simulink model "simulator_model"  (R2016a)
settings: Solver=FixedStepAuto  StartTime=0.0  StopTime=30  FixedStep=0.1  RelTol=1e-3
model workspace: external: MAT-File /home/combine/bin/ExjobbROV/simulink/Estimation/parameters.mat (data not in the file)
libraries: simulink x10, dspsrcs4 x6
settings Model: SimulationMode=accelerator  Creator=erik  LastModifiedBy=combine
settings DataIOCC: LimitDataPoints=on  InspectSignalLogs=on
settings OptimizationCC: EfficientMapNaN2IntZero=off
settings DebuggingCC: AllowSymbolicDim=off
settings HardwareCC: TargetBitPerLong=64  TargetBitPerPointer=64  TargetLongLongMode=on  TargetIntDivRoundTo=Zero  TargetEndianess=LittleEndian  TargetWordSize=64  TargetHWDeviceType=MATLAB Host  ProdEqTarget=off
settings ModelReferenceCC: PropagateSignalLabelsOutOfModel=off
settings CodeAppCC: MaxIdLength=128
settings GRTTargetCC: GeneratePreprocessorConditionals=Use local settings  CombineOutputUpdateFcns=off  GRTInterface=on

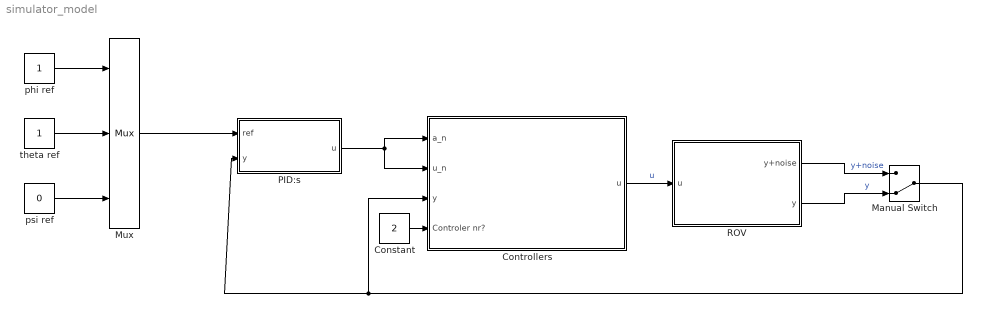
== system simulator_model ==
  Constant : Constant  Value=2
  Controllers : Subsystem
  Manual Switch : ManualSwitch  CurrentSetting=0
  Mux : Mux  Inputs=3
  PID:s : Subsystem
  ROV : Subsystem
  phi ref : Constant
  "psi ref " : Constant  Value=0
  "theta ref " : Constant
  wires:
  Controllers/1(u) -> ROV/1(u)  "u"
  Constant/1 -> Controllers/4(Controler nr?)
  ROV/2(y) -> Manual Switch/2  "y"
  ROV/1(y+noise) -> Manual Switch/1  "y+noise"
  Manual Switch/1 -> PID:s/2(y), Controllers/3(y)
  PID:s/1(u) -> Controllers/2(u_n), Controllers/1(a_n)
  phi ref/1 -> Mux/1
  "theta ref "/1 -> Mux/2
  "psi ref "/1 -> Mux/3
  Mux/1 -> PID:s/1(ref)

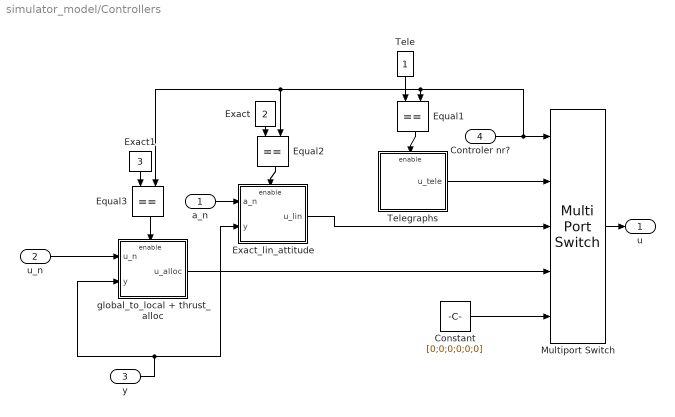
== system simulator_model/Controllers ==
  a_n : Inport
  u_n : Inport  Port=2
  y : Inport  Port=3
  Controler nr? : Inport  Port=4
  Constant : Constant  Value=[0;0;0;0;0;0]
  Equal1 : RelationalOperator  Operator===  OutDataTypeStr=boolean
  Equal2 : RelationalOperator  Operator===  OutDataTypeStr=boolean
  Equal3 : RelationalOperator  Operator===  OutDataTypeStr=boolean
  Exact : Constant  Value=2
  Exact1 : Constant  Value=3
  Exact_lin_attitude : Subsystem
  Multiport Switch : MultiPortSwitch  Inputs=4
  Tele : Constant
  Telegraphs : Subsystem
  global_to_local + thrust_alloc : Subsystem
  u : Outport
  wires:
  Exact1/1 -> Equal3/1
  Multiport Switch/1 -> u/1
  Constant/1 -> Multiport Switch/5
  Telegraphs/1(u_tele) -> Multiport Switch/2
  Exact_lin_attitude/1(u_lin) -> Multiport Switch/3
  global_to_local + thrust_alloc/1(u_alloc) -> Multiport Switch/4
  Controler nr?/1 -> Multiport Switch/1, Equal1/2, Equal2/2, Equal3/2
  Equal1/1 -> Telegraphs/Enable
  Tele/1 -> Equal1/1
  Exact/1 -> Equal2/1
  Equal2/1 -> Exact_lin_attitude/Enable
  Equal3/1 -> global_to_local + thrust_alloc/Enable
  y/1 -> Exact_lin_attitude/2(y), global_to_local + thrust_alloc/2(y)
  u_n/1 -> global_to_local + thrust_alloc/1(u_n)
  a_n/1 -> Exact_lin_attitude/1(a_n)

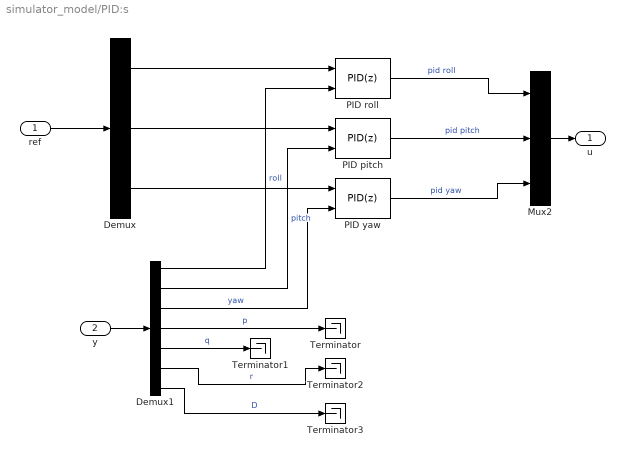
== system simulator_model/PID:s ==
  ref : Inport
  y : Inport  Port=2
  Demux : Demux  Outputs=3
  Demux1 : Demux  Outputs=7
  Mux2 : Mux  Inputs=3
  PID pitch : simulink/Continuous/PID Controller (2DOF)  Controller=PID  TimeDomain=Discrete-time  SampleTime=-1  IntegratorMethod=Forward Euler  FilterMethod=Forward Euler  Form=Parallel  UseFilter=on  ControllerParametersSource=internal  P=1  I=1  D=0  N=1  b=1  c=1  InitialConditionSource=internal  InitialConditionForIntegrator=0  InitialConditionForFilter=0  ExternalReset=none  LimitOutput=off  UpperSaturationLimit=inf  LowerSaturationLimit=-inf  LinearizeAsGain=on  AntiWindupMode=none  Kb=1  TrackingMode=off  Kt=1  PParamMin=[]  PParamMax=[]  IParamMin=[]  IParamMax=[]  DParamMin=[]  DParamMax=[]  NParamMin=[]  NParamMax=[]  bParamMin=[]  bParamMax=[]  cParamMin=[]  cParamMax=[]  KbParamMin=[]  KbParamMax=[]  KtParamMin=[]  KtParamMax=[]  POutMin=[]  POutMax=[]  IOutMin=[]  IOutMax=[]  DOutMin=[]  DOutMax=[]  NOutMin=[]  NOutMax=[]  bOutMin=[]  bOutMax=[]  cOutMin=[]  cOutMax=[]  KbOutMin=[]  KbOutMax=[]  KtOutMin=[]  KtOutMax=[]  IntegratorOutMin=[]  IntegratorOutMax=[]  FilterOutMin=[]  FilterOutMax=[]  SumOutMin=[]  SumOutMax=[]  Sum1OutMin=[]  Sum1OutMax=[]  Sum2OutMin=[]  Sum2OutMax=[]  Sum3OutMin=[]  Sum3OutMax=[]  SumI1OutMin=[]  SumI1OutMax=[]  SumI2OutMin=[]  SumI2OutMax=[]  SumI3OutMin=[]  SumI3OutMax=[]  SumDOutMin=[]  SumDOutMax=[]  SaturationOutMin=[]  SaturationOutMax=[]  IntegratorContinuousStateAttributes=''  IntegratorStateMustResolveToSignalObject=off  IntegratorRTWStateStorageClass=Auto  FilterContinuousStateAttributes=''  FilterStateMustResolveToSignalObject=off  FilterRTWStateStorageClass=Auto  DifferentiatorICPrevScaledInput=0  DifferentiatorOutMin=[]  DifferentiatorOutMax=[]
  PID roll : simulink/Continuous/PID Controller (2DOF)  Controller=PID  TimeDomain=Discrete-time  SampleTime=-1  IntegratorMethod=Forward Euler  FilterMethod=Forward Euler  Form=Parallel  UseFilter=on  ControllerParametersSource=internal  P=1  I=1  D=0  N=1  b=1  c=1  InitialConditionSource=internal  InitialConditionForIntegrator=0  InitialConditionForFilter=0  ExternalReset=none  LimitOutput=off  UpperSaturationLimit=inf  LowerSaturationLimit=-inf  LinearizeAsGain=on  AntiWindupMode=none  Kb=1  TrackingMode=off  Kt=1  PParamMin=[]  PParamMax=[]  IParamMin=[]  IParamMax=[]  DParamMin=[]  DParamMax=[]  NParamMin=[]  NParamMax=[]  bParamMin=[]  bParamMax=[]  cParamMin=[]  cParamMax=[]  KbParamMin=[]  KbParamMax=[]  KtParamMin=[]  KtParamMax=[]  POutMin=[]  POutMax=[]  IOutMin=[]  IOutMax=[]  DOutMin=[]  DOutMax=[]  NOutMin=[]  NOutMax=[]  bOutMin=[]  bOutMax=[]  cOutMin=[]  cOutMax=[]  KbOutMin=[]  KbOutMax=[]  KtOutMin=[]  KtOutMax=[]  IntegratorOutMin=[]  IntegratorOutMax=[]  FilterOutMin=[]  FilterOutMax=[]  SumOutMin=[]  SumOutMax=[]  Sum1OutMin=[]  Sum1OutMax=[]  Sum2OutMin=[]  Sum2OutMax=[]  Sum3OutMin=[]  Sum3OutMax=[]  SumI1OutMin=[]  SumI1OutMax=[]  SumI2OutMin=[]  SumI2OutMax=[]  SumI3OutMin=[]  SumI3OutMax=[]  SumDOutMin=[]  SumDOutMax=[]  SaturationOutMin=[]  SaturationOutMax=[]  IntegratorContinuousStateAttributes=''  IntegratorStateMustResolveToSignalObject=off  IntegratorRTWStateStorageClass=Auto  FilterContinuousStateAttributes=''  FilterStateMustResolveToSignalObject=off  FilterRTWStateStorageClass=Auto  DifferentiatorICPrevScaledInput=0  DifferentiatorOutMin=[]  DifferentiatorOutMax=[]
  PID yaw : simulink/Continuous/PID Controller (2DOF)  Controller=PID  TimeDomain=Discrete-time  SampleTime=-1  IntegratorMethod=Forward Euler  FilterMethod=Forward Euler  Form=Parallel  UseFilter=on  ControllerParametersSource=internal  P=0  I=0  D=0  N=1  b=1  c=1  InitialConditionSource=internal  InitialConditionForIntegrator=0  InitialConditionForFilter=0  ExternalReset=none  LimitOutput=off  UpperSaturationLimit=inf  LowerSaturationLimit=-inf  LinearizeAsGain=on  AntiWindupMode=none  Kb=1  TrackingMode=off  Kt=1  PParamMin=[]  PParamMax=[]  IParamMin=[]  IParamMax=[]  DParamMin=[]  DParamMax=[]  NParamMin=[]  NParamMax=[]  bParamMin=[]  bParamMax=[]  cParamMin=[]  cParamMax=[]  KbParamMin=[]  KbParamMax=[]  KtParamMin=[]  KtParamMax=[]  POutMin=[]  POutMax=[]  IOutMin=[]  IOutMax=[]  DOutMin=[]  DOutMax=[]  NOutMin=[]  NOutMax=[]  bOutMin=[]  bOutMax=[]  cOutMin=[]  cOutMax=[]  KbOutMin=[]  KbOutMax=[]  KtOutMin=[]  KtOutMax=[]  IntegratorOutMin=[]  IntegratorOutMax=[]  FilterOutMin=[]  FilterOutMax=[]  SumOutMin=[]  SumOutMax=[]  Sum1OutMin=[]  Sum1OutMax=[]  Sum2OutMin=[]  Sum2OutMax=[]  Sum3OutMin=[]  Sum3OutMax=[]  SumI1OutMin=[]  SumI1OutMax=[]  SumI2OutMin=[]  SumI2OutMax=[]  SumI3OutMin=[]  SumI3OutMax=[]  SumDOutMin=[]  SumDOutMax=[]  SaturationOutMin=[]  SaturationOutMax=[]  IntegratorContinuousStateAttributes=''  IntegratorStateMustResolveToSignalObject=off  IntegratorRTWStateStorageClass=Auto  FilterContinuousStateAttributes=''  FilterStateMustResolveToSignalObject=off  FilterRTWStateStorageClass=Auto  DifferentiatorICPrevScaledInput=0  DifferentiatorOutMin=[]  DifferentiatorOutMax=[]
  Terminator{,1..3} (4 alike) : Terminator
  u : Outport
  wires:
  Mux2/1 -> u/1
  Demux1/1 -> PID roll/2  "roll"
  Demux1/2 -> PID pitch/2  "pitch"
  Demux1/3 -> PID yaw/2  "yaw"
  Demux/2 -> PID pitch/1
  PID pitch/1 -> Mux2/2  "pid pitch"
  Demux/1 -> PID roll/1
  PID roll/1 -> Mux2/1  "pid roll"
  PID yaw/1 -> Mux2/3  "pid yaw"
  Demux/3 -> PID yaw/1
  y/1 -> Demux1/1
  ref/1 -> Demux/1
  Demux1/4 -> Terminator/1  "p"
  Demux1/5 -> Terminator1/1  "q"
  Demux1/6 -> Terminator2/1  "r"
  Demux1/7 -> Terminator3/1  "D"

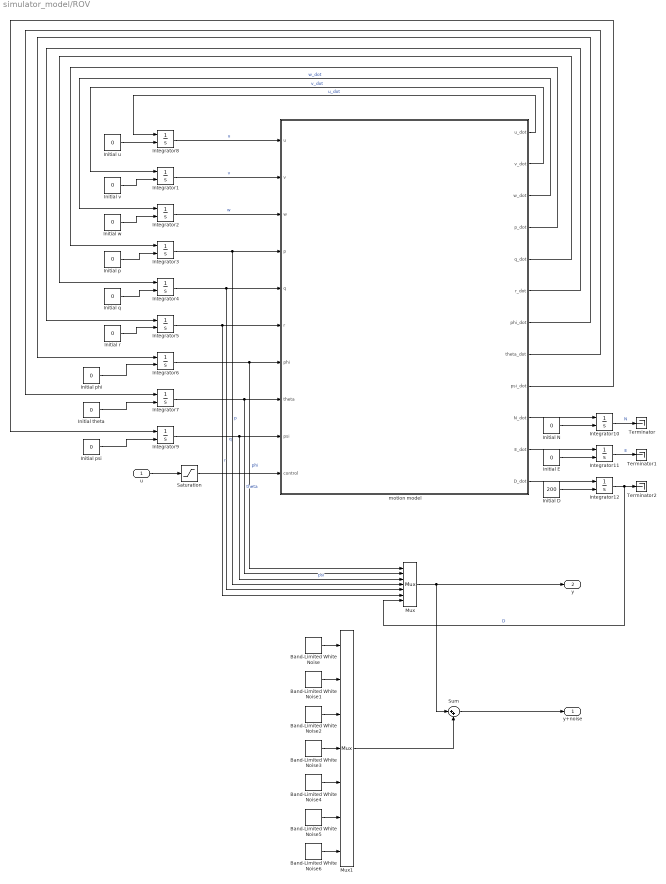
== system simulator_model/ROV ==
  u : Inport
  Band-Limited White Noise : simulink/Sources/Band-Limited White Noise  Cov=0.0005  Ts=0.1  seed=[23341]
  Band-Limited White Noise1 : simulink/Sources/Band-Limited White Noise  Cov=0.0005  Ts=0.1  seed=[29023]
  Band-Limited White Noise2 : simulink/Sources/Band-Limited White Noise  Cov=0.0005  Ts=0.1  seed=[91318]
  Band-Limited White Noise3 : simulink/Sources/Band-Limited White Noise  Cov=0.0005  Ts=0.1  seed=[2333451]
  Band-Limited White Noise4 : simulink/Sources/Band-Limited White Noise  Cov=0.0005  Ts=0.1  seed=[21241]
  Band-Limited White Noise5 : simulink/Sources/Band-Limited White Noise  Cov=0.0005  Ts=0.1  seed=[12345]
  Band-Limited White Noise6 : simulink/Sources/Band-Limited White Noise  Cov=0.0005  Ts=0.1  seed=[9875]
  Initial D : Constant  Value=200
  Initial E : Constant  Value=0
  Initial N : Constant  Value=0
  Initial p : Constant  Value=0
  Initial phi : Constant  Value=0
  Initial psi : Constant  Value=0
  Initial q : Constant  Value=0
  Initial r : Constant  Value=0
  Initial theta : Constant  Value=0
  Initial u : Constant  Value=0
  Initial v : Constant  Value=0
  Initial w : Constant  Value=0
  Integrator{1..12} (12 alike) : Integrator  InitialConditionSource=external
  Mux : Mux  Inputs=7
  Mux1 : Mux  Inputs=7
  Saturation : Saturate  UpperLimit=1  LowerLimit=-1
  Sum : Sum  Inputs=|++
  Terminator : Terminator
  Terminator1 : Terminator
  Terminator2 : Terminator
  motion model : MATLAB Function  TreatAsAtomicUnit=on
  y+noise : Outport  PortDimensions=7
  y : Outport  Port=2  PortDimensions=7
  wires:
  u/1 -> Saturation/1
  Integrator8/1 -> motion model/1(u)  "u"
  Integrator1/1 -> motion model/2(v)  "v"
  Integrator2/1 -> motion model/3(w)  "w"
  Integrator3/1 -> Mux/4, motion model/4(p)  "p"
  Integrator4/1 -> Mux/5, motion model/5(q)  "q"
  Integrator5/1 -> Mux/6, motion model/6(r)  "r"
  Integrator7/1 -> Mux/2, motion model/8(theta)  "theta"
  Integrator9/1 -> Mux/3, motion model/9(psi)  "psi"
  motion model/1(u_dot) -> Integrator8/1  "u_dot"
  motion model/2(v_dot) -> Integrator1/1  "v_dot"
  motion model/3(w_dot) -> Integrator2/1  "w_dot"
  motion model/4(p_dot) -> Integrator3/1
  motion model/5(q_dot) -> Integrator4/1
  motion model/6(r_dot) -> Integrator5/1
  motion model/7(phi_dot) -> Integrator6/1
  motion model/8(theta_dot) -> Integrator7/1
  motion model/9(psi_dot) -> Integrator9/1
  Initial u/1 -> Integrator8/2
  Initial v/1 -> Integrator1/2
  Initial w/1 -> Integrator2/2
  Initial p/1 -> Integrator3/2
  Initial q/1 -> Integrator4/2
  Initial r/1 -> Integrator5/2
  Initial phi/1 -> Integrator6/2
  Integrator6/1 -> Mux/1, motion model/7(phi)  "phi"
  Initial theta/1 -> Integrator7/2
  Initial psi/1 -> Integrator9/2
  motion model/10(N_dot) -> Integrator10/1
  motion model/11(E_dot) -> Integrator11/1
  motion model/12(D_dot) -> Integrator12/1
  Initial E/1 -> Integrator11/2
  Initial N/1 -> Integrator10/2
  Initial D/1 -> Integrator12/2
  Integrator10/1 -> Terminator/1  "N"
  Integrator11/1 -> Terminator1/1  "E"
  Integrator12/1 -> Mux/7, Terminator2/1  "D"
  Mux/1 -> Sum/1, y/1
  Sum/1 -> y+noise/1
  Saturation/1 -> motion model/10(control)
  Band-Limited White Noise/1 -> Mux1/1
  Band-Limited White Noise1/1 -> Mux1/2
  Band-Limited White Noise2/1 -> Mux1/3
  Band-Limited White Noise3/1 -> Mux1/4
  Band-Limited White Noise4/1 -> Mux1/5
  Band-Limited White Noise5/1 -> Mux1/6
  Band-Limited White Noise6/1 -> Mux1/7
  Mux1/1 -> Sum/2

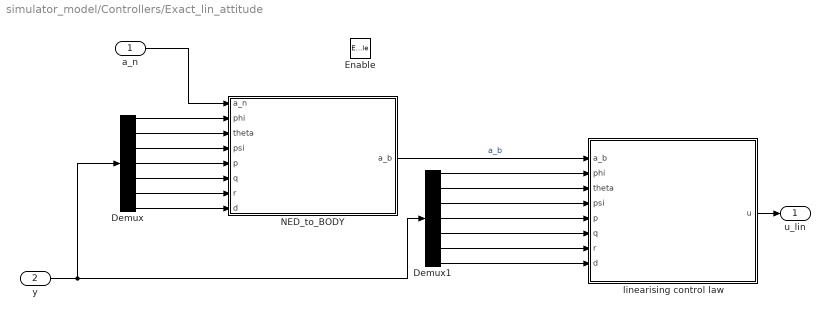
== system simulator_model/Controllers/Exact_lin_attitude ==
  a_n : Inport  PortDimensions=3
  y : Inport  Port=2  PortDimensions=7
  Enable : EnablePort
  Demux : Demux  Outputs=7
  Demux1 : Demux  Outputs=7
  NED_to_BODY : MATLAB Function  TreatAsAtomicUnit=on
  linearising control law : MATLAB Function  TreatAsAtomicUnit=on
  u_lin : Outport  PortDimensions=6
  wires:
  linearising control law/1(u) -> u_lin/1
  a_n/1 -> NED_to_BODY/1(a_n)
  NED_to_BODY/1(a_b) -> linearising control law/1(a_b)  "a_b"
  y/1 -> Demux1/1, Demux/1
  Demux/6 -> NED_to_BODY/7(r)
  Demux/4 -> NED_to_BODY/5(p)
  Demux/7 -> NED_to_BODY/8(d)
  Demux/1 -> NED_to_BODY/2(phi)
  Demux/3 -> NED_to_BODY/4(psi)
  Demux/5 -> NED_to_BODY/6(q)
  Demux/2 -> NED_to_BODY/3(theta)
  Demux1/1 -> linearising control law/2(phi)
  Demux1/2 -> linearising control law/3(theta)
  Demux1/3 -> linearising control law/4(psi)
  Demux1/4 -> linearising control law/5(p)
  Demux1/5 -> linearising control law/6(q)
  Demux1/6 -> linearising control law/7(r)
  Demux1/7 -> linearising control law/8(d)

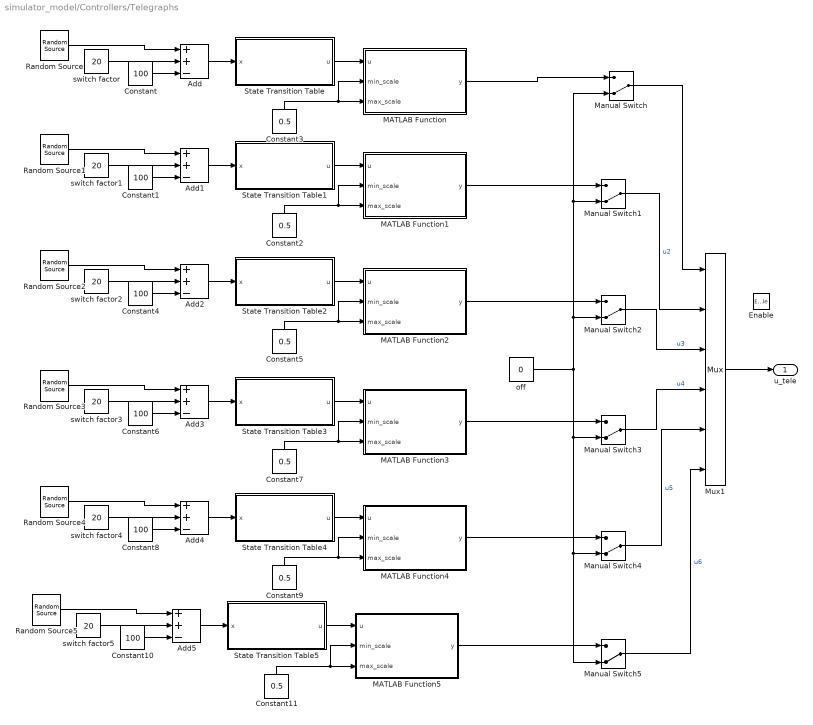
== system simulator_model/Controllers/Telegraphs ==
  Enable : EnablePort
  Add{,1..5} (6 alike) : Sum  Inputs=++-
  Constant{,1,4,6,8,10} (6 alike) : Constant  Value=100
  Constant{2..3,5,7,9,11} (6 alike) : Constant  Value=0.5
  MATLAB Function : MATLAB Function  TreatAsAtomicUnit=on
  MATLAB Function1 : MATLAB Function  TreatAsAtomicUnit=on
  MATLAB Function2 : MATLAB Function  TreatAsAtomicUnit=on
  MATLAB Function3 : MATLAB Function  TreatAsAtomicUnit=on
  MATLAB Function4 : MATLAB Function  TreatAsAtomicUnit=on
  MATLAB Function5 : MATLAB Function  TreatAsAtomicUnit=on
  Manual Switch{,1..5} (6 alike) : ManualSwitch  CurrentSetting=0
  Mux1 : Mux  Inputs=6
  Random Source{,1..5} (6 alike) : dspsrcs4/Random Source  SrcType=Uniform  NormMethod=Ziggurat  CltLength=12  MinVal=1  MaxVal=100  MeanVal=0  VarVal=1  RepMode=Not repeatable  rawSeed=1  IsInherit=on  SampMode=Discrete  SampTime=0.1  SampFrame=1  DataType=Double  OutComplex=Real  OutputFrames=off
  State Transition Table : State Transition Table  TreatAsAtomicUnit=on
  State Transition Table1 : State Transition Table  TreatAsAtomicUnit=on
  State Transition Table2 : State Transition Table  TreatAsAtomicUnit=on
  State Transition Table3 : State Transition Table  TreatAsAtomicUnit=on
  State Transition Table4 : State Transition Table  TreatAsAtomicUnit=on
  State Transition Table5 : State Transition Table  TreatAsAtomicUnit=on
  off : Constant  Value=0
  switch factor{,1..5} (6 alike) : Constant  Value=20
  u_tele : Outport
  wires:
  Random Source/1 -> Add/1
  Constant/1 -> Add/3
  Add/1 -> State Transition Table/1(x)
  switch factor/1 -> Add/2
  State Transition Table/1(u) -> MATLAB Function/1(u)
  Constant3/1 -> MATLAB Function/3(max_scale), MATLAB Function/2(min_scale)
  Random Source1/1 -> Add1/1
  Constant1/1 -> Add1/3
  Add1/1 -> State Transition Table1/1(x)
  switch factor1/1 -> Add1/2
  State Transition Table1/1(u) -> MATLAB Function1/1(u)
  Constant2/1 -> MATLAB Function1/3(max_scale), MATLAB Function1/2(min_scale)
  Random Source2/1 -> Add2/1
  Constant4/1 -> Add2/3
  Add2/1 -> State Transition Table2/1(x)
  switch factor2/1 -> Add2/2
  State Transition Table2/1(u) -> MATLAB Function2/1(u)
  Constant5/1 -> MATLAB Function2/3(max_scale), MATLAB Function2/2(min_scale)
  Random Source3/1 -> Add3/1
  Constant6/1 -> Add3/3
  Add3/1 -> State Transition Table3/1(x)
  switch factor3/1 -> Add3/2
  State Transition Table3/1(u) -> MATLAB Function3/1(u)
  Constant7/1 -> MATLAB Function3/3(max_scale), MATLAB Function3/2(min_scale)
  Random Source4/1 -> Add4/1
  Constant8/1 -> Add4/3
  Add4/1 -> State Transition Table4/1(x)
  switch factor4/1 -> Add4/2
  State Transition Table4/1(u) -> MATLAB Function4/1(u)
  Constant9/1 -> MATLAB Function4/3(max_scale), MATLAB Function4/2(min_scale)
  Random Source5/1 -> Add5/1
  Constant10/1 -> Add5/3
  Add5/1 -> State Transition Table5/1(x)
  switch factor5/1 -> Add5/2
  State Transition Table5/1(u) -> MATLAB Function5/1(u)
  Constant11/1 -> MATLAB Function5/3(max_scale), MATLAB Function5/2(min_scale)
  MATLAB Function/1(y) -> Manual Switch/1
  MATLAB Function1/1(y) -> Manual Switch1/1
  MATLAB Function2/1(y) -> Manual Switch2/1
  MATLAB Function3/1(y) -> Manual Switch3/1
  MATLAB Function4/1(y) -> Manual Switch4/1
  MATLAB Function5/1(y) -> Manual Switch5/1
  off/1 -> Manual Switch1/2, Manual Switch/2, Manual Switch2/2, Manual Switch5/2, Manual Switch4/2, Manual Switch3/2
  Manual Switch/1 -> Mux1/1
  Manual Switch1/1 -> Mux1/2  "u2"
  Manual Switch2/1 -> Mux1/3  "u3"
  Manual Switch3/1 -> Mux1/4  "u4"
  Manual Switch4/1 -> Mux1/5  "u5"
  Manual Switch5/1 -> Mux1/6  "u6"
  Mux1/1 -> u_tele/1

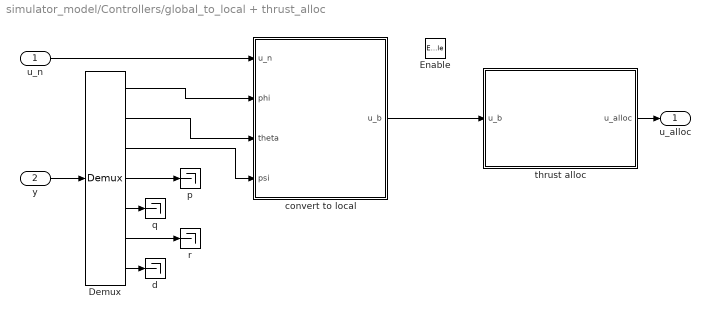
== system simulator_model/Controllers/global_to_local + thrust_alloc ==
  u_n : Inport
  y : Inport  Port=2
  Enable : EnablePort
  Demux : Demux  Outputs=7
  convert to local : MATLAB Function  TreatAsAtomicUnit=on
  d : Terminator
  p : Terminator
  q : Terminator
  r : Terminator
  thrust alloc : MATLAB Function  TreatAsAtomicUnit=on
  u_alloc : Outport
  wires:
  convert to local/1(u_b) -> thrust alloc/1(u_b)
  y/1 -> Demux/1
  Demux/1 -> convert to local/2(phi)
  Demux/2 -> convert to local/3(theta)
  Demux/3 -> convert to local/4(psi)
  Demux/4 -> p/1
  Demux/5 -> q/1
  Demux/6 -> r/1
  Demux/7 -> d/1
  u_n/1 -> convert to local/1(u_n)
  thrust alloc/1(u_alloc) -> u_alloc/1

== matlab function simulator_model/Controllers/Telegraphs/MATLAB Function ==
  data: u input; y output; min_scale input; max_scale input
function y = fcn(u, min_scale, max_scale)
%#codegen
    if (u < 0)
        y = min_scale*u;
    else
        y = max_scale*u;
    end
end

== matlab function simulator_model/ROV/motion model ==
  data: u input; u_dot output; v input; w input; p input; q input; r input; phi input; theta input; psi input; control input; v_dot output; w_dot output; p_dot output; q_dot output; r_dot output; phi_dot output; theta_dot output; psi_dot output; N_dot output; E_dot output; D_dot output; parameters parameter
function [u_dot, v_dot, w_dot, p_dot, q_dot, r_dot, phi_dot, theta_dot, psi_dot, N_dot, E_dot, D_dot] =...
    fcn(u, v, w, p, q, r, phi, theta, psi,control,parameters)
%#codegen
cphi=cos(phi);
cth=cos(theta);
cpsi=cos(psi);

sphi=sin(phi);
sth=sin(theta);
spsi=sin(psi);

u1 = control(1);
u2 = control(2);
u3 = control(3);
u4 = control(4);
u5 = control(5);
u6 = control(6);




lookup =[...
  -40.0337   -1.0000
  -40.0337   -0.9750
  -40.0788   -0.9500
  -37.5428   -0.9250
  -36.6092   -0.9000
  -35.4971   -0.8750
  -33.7623   -0.8500
  -32.3835   -0.8250
  -31.2263   -0.8000
  -29.9809   -0.7750
  -28.5128   -0.7500
  -27.6234   -0.7250
  -26.5554   -0.7000
  -24.7765   -0.6750
  -23.1751   -0.6500
  -22.1522   -0.6250
  -21.3510   -0.6000
  -19.5280   -0.5750
  -18.4600   -0.5500
  -17.3480   -0.5250
  -16.1025   -0.5000
  -14.6345   -0.4750
  -13.0781   -0.4500
  -12.1877   -0.4250
  -10.9874   -0.4000
  -10.0528   -0.3750
   -8.8966   -0.3500
   -7.7404   -0.3250
   -6.8058   -0.3000
   -6.0497   -0.2750
   -5.1151   -0.2500
   -4.2698   -0.2250
   -3.4696   -0.2000
   -2.7135   -0.1750
   -1.8682   -0.1500
   -1.1121   -0.1250
   -0.5335   -0.1000
   -0.2667   -0.0750
         0   -0.0500
         0   -0.0250
         0         0
         0    0.0250
         0    0.0500
    0.5786    0.0750
    1.1121    0.1000
    1.8240    0.1250
    2.5801    0.1500
    3.4255    0.1750
    4.0923    0.2000
    5.1151    0.2250
    6.2272    0.2500
    7.0284    0.2750
    8.2739    0.3000
    9.2526    0.3250
   10.8089    0.3500
   12.2328    0.3750
   13.6558    0.4000
   14.9904    0.4250
   16.4585    0.4500
   17.7039    0.4750
   19.2161    0.5000
   20.5508    0.5250
   21.7521    0.5500
   23.6644    0.5750
   24.7324    0.6000
   26.4221    0.6250
   27.7126    0.6500
   29.6249    0.6750
   31.3156    0.7000
   32.8729    0.7250
   33.8065    0.7500
   34.2517    0.7750
   37.0534    0.8000
   38.6549    0.8250
   39.2776    0.8500
   41.1458    0.8750
   42.9257    0.9000
   44.7938    0.9250
   47.1062    0.9500
   48.0408    0.9750
   49.9531    1.0000];


%Thrustherforce in newtons.

 f1 = interp1(lookup(:,2),lookup(:,1),u1);
 f2 = interp1(lookup(:,2),lookup(:,1),u2);
 f3 = interp1(lookup(:,2),lookup(:,1),u3);
 f4 = interp1(lookup(:,2),lookup(:,1),u4);
 f5 = interp1(lookup(:,2),lookup(:,1),u5);
 f6 = interp1(lookup(:,2),lookup(:,1),u6);

%Parameters that are not given by estimation
%%%%%%%%%%%%%%
Xu  = -0.1;
Xu_dot  = -0.1;
Xu_abs_u  = -0.1;

Yv  = -0.3;
Yv_dot  = -0.3;
Yv_abs_v  = -0.3;

Zw  = -0.4;
Zw_dot  = -0.4;
Zw_abs_w  = -0.4;
%%%%%%%%%%%
%Estimated parameters. Load from param array
m = parameters(1);
g = parameters(2);
rho = parameters(3);
V = parameters(4);
 %Thruster placement from CO [m]
lx1 = parameters(5);
ly1 = parameters(6);
ly2 = parameters(7);
lx2 = parameters(8);
ly3 = parameters(9);
lx5 = parameters(10);
ly4 = parameters(11);
lz6 = parameters(12);
zb = parameters(13);
Xu = parameters(14);
Xu_dot = parameters(15);
Xu_abs_u = parameters(16);
Yv = parameters(17);
Yv_dot = parameters(18);
Yv_abs_v = parameters(19);
Zw = parameters(20);
Zw_dot = parameters(21);
Zw_abs_w = parameters(22);
Kp = parameters(23);
Kp_dot = parameters(24);
Kp_abs_p = parameters(25);
Mq = parameters(26);
Mq_dot = parameters(27);
Mq_abs_q = parameters(28);
Nr = parameters(29);
Nr_dot = parameters(30);
Nr_abs_r = parameters(31);
Ix = parameters(32);
Iy = parameters(33);
Iz = parameters(34);
B = rho*g*V;
W = m*g;


%Full model
%Observe that parameters unique to u, v and w cannot be estimated at the
%present time. Placeholder values are used for simulation.
u_dot =...
    -(f3 + f4 + u*(Xu + Xu_abs_u*abs(u)) + sth*(B - W) - m*(q*w - r*v) - Yv_dot*r*v + Zw_dot*q*w)/(Xu_dot - m);
 
 
v_dot =...
    (f6 - v*(Yv + Yv_abs_v*abs(v)) - m*(p*w - r*u) + cth*sphi*(B - W) - Xu_dot*r*u + Zw_dot*p*w)/(Yv_dot - m);
 
 
w_dot =...
    (f1 + f2 + f5 - w*(Zw + Zw_abs_w*abs(w)) + m*(p*v - q*u) + cphi*cth*(B - W) + Xu_dot*q*u - Yv_dot*p*v)/(Zw_dot - m);
 
 
p_dot =...
    (f1*ly1 - f2*ly2 + f6*lz6 + p*(Kp + Kp_abs_p*abs(p)) - Mq_dot*q*r + Nr_dot*q*r + q*r*(Iy - Iz) - Yv_dot*v*w + Zw_dot*v*w + B*cth*sphi*zb)/(Ix - Kp_dot);
 
 
q_dot =...
    (f1*lx1 + f2*lx2 - f5*lx5 + q*(Mq + Mq_abs_q*abs(q)) + Kp_dot*p*r + B*sth*zb - Nr_dot*p*r - p*r*(Ix - Iz) + Xu_dot*u*w - Zw_dot*u*w)/(Iy - Mq_dot);
 
 
r_dot =...
    (r*(Nr + Nr_abs_r*abs(r)) + f3*ly3 - f4*ly4 - Kp_dot*p*q + Mq_dot*p*q + p*q*(Ix - Iy) - Xu_dot*u*v + Yv_dot*u*v)/(Iz - Nr_dot);
 
    
N_dot     =  u*(cpsi*cth) +   v*(-spsi*cphi+cpsi*sth*sphi)    +   w*(spsi*sphi+cpsi*cphi*sth);
E_dot     =  u*(spsi*cth) +   v*(cpsi*cphi+sphi*sth*spsi)     +   w*(-cpsi*sphi+sth*spsi*cphi);
D_dot     =  u*(-sth)     +   v*(cth*sphi)                    +   w*(cth*cphi);


phi_dot     =   p + q*sphi*sth/cth + r*cphi*sth/cth;
theta_dot   =   q*cphi - r*sphi;
psi_dot     =   q*sphi/cth   +   r*cphi/cth;
end

== matlab function simulator_model/Controllers/Telegraphs/MATLAB Function1 ==
  data: u input; y output; min_scale input; max_scale input
function y = fcn(u,min_scale,max_scale)
%#codegen
    
    if (u < 0)
        y = min_scale*u;
    else
        y = max_scale*u;
    end
end

== stateflow chart simulator_model/Controllers/Telegraphs/State Transition Table1 ==
  state state1
  state state2
  (default) -> state1
  state1 -> (junction 20) [order 2]
  (junction 20) -> state1
  state1 -> state2 [order 1] : [x > 0]
      | {u = 1}
  state2 -> state1 [order 1] : [x> 0]
      | {u= -1}
  state2 -> (junction 24) [order 2]
  (junction 24) -> state2
  data: x input; u output

== matlab function simulator_model/Controllers/Telegraphs/MATLAB Function2 ==
  data: u input; y output; min_scale input; max_scale input
function y = fcn(u,min_scale,max_scale)
%#codegen
    
    if (u < 0)
        y = min_scale*u;
    else
        y = max_scale*u;
    end
end

== stateflow chart simulator_model/Controllers/Telegraphs/State Transition Table ==
  state state1
  state state2
  (default) -> state1
  state1 -> (junction 20) [order 2]
  (junction 20) -> state1
  state1 -> state2 [order 1] : [x > 0]
      | {u = 1}
  state2 -> state1 [order 1] : [x> 0]
      | {u= -1}
  state2 -> (junction 24) [order 2]
  (junction 24) -> state2
  data: x input; u output

== stateflow chart simulator_model/Controllers/Telegraphs/State Transition Table2 ==
  state state1
  state state2
  (default) -> state1
  state1 -> (junction 20) [order 2]
  (junction 20) -> state1
  state1 -> state2 [order 1] : [x > 0]
      | {u = 1}
  state2 -> state1 [order 1] : [x> 0]
      | {u= -1}
  state2 -> (junction 24) [order 2]
  (junction 24) -> state2
  data: x input; u output

== matlab function simulator_model/Controllers/Telegraphs/MATLAB Function3 ==
  data: u input; y output; min_scale input; max_scale input
function y = fcn(u,min_scale,max_scale)
%#codegen
    
    if (u < 0)
        y = min_scale*u;
    else
        y = max_scale*u;
    end
end

== stateflow chart simulator_model/Controllers/Telegraphs/State Transition Table3 ==
  state state1
  state state2
  (default) -> state1
  state1 -> (junction 20) [order 2]
  (junction 20) -> state1
  state1 -> state2 [order 1] : [x > 0]
      | {u = 1}
  state2 -> state1 [order 1] : [x> 0]
      | {u= -1}
  state2 -> (junction 24) [order 2]
  (junction 24) -> state2
  data: x input; u output

== matlab function simulator_model/Controllers/Telegraphs/MATLAB Function4 ==
  data: u input; y output; min_scale input; max_scale input
function y = fcn(u,min_scale,max_scale)
%#codegen
    
    if (u < 0)
        y = min_scale*u;
    else
        y = max_scale*u;
    end
end

== stateflow chart simulator_model/Controllers/Telegraphs/State Transition Table4 ==
  state state1
  state state2
  (default) -> state1
  state1 -> (junction 20) [order 2]
  (junction 20) -> state1
  state1 -> state2 [order 1] : [x > 0]
      | {u = 1}
  state2 -> state1 [order 1] : [x> 0]
      | {u= -1}
  state2 -> (junction 24) [order 2]
  (junction 24) -> state2
  data: x input; u output

== matlab function simulator_model/Controllers/Telegraphs/MATLAB Function5 ==
  data: u input; y output; min_scale input; max_scale input
function y = fcn(u,min_scale,max_scale)
%#codegen
    
    if (u < 0)
        y = min_scale*u;
    else
        y = max_scale*u;
    end
end

== stateflow chart simulator_model/Controllers/Telegraphs/State Transition Table5 ==
  state state1
  state state2
  (default) -> state1
  state1 -> (junction 20) [order 2]
  (junction 20) -> state1
  state1 -> state2 [order 1] : [x > 0]
      | {u = 1}
  state2 -> state1 [order 1] : [x> 0]
      | {u= -1}
  state2 -> (junction 24) [order 2]
  (junction 24) -> state2
  data: x input; u output

== matlab function simulator_model/Controllers/global_to_local + thrust_alloc/convert to local ==
  data: u_n input; u_b output size=6; phi input; theta input; psi input
function u_b = global_to_local(u_n,phi,theta,psi)
%#codegen
sphi = sin(phi);
cphi = cos(phi);
spsi = sin(psi);
cpsi = cos(psi);
sth = sin(theta);
cth = cos(theta);
R= ([...
    cpsi*cth, -spsi*cphi+cpsi*sth*sphi, spsi*sphi+cpsi*cphi*sth;
    spsi*cth, cpsi*cphi+sphi*sth*spsi, -cpsi*sphi+sth*spsi*cphi;
    -sth, cth*sphi, cth*cphi]);
rotmatrix = blkdiag(R,R);

u_b=rotmatrix*[0;0;0;u_n];
end

== matlab function simulator_model/Controllers/Exact_lin_attitude/NED_to_BODY ==
  data: a_n input; phi input; theta input; psi input; a_b output size=3; p input; q input; r input; d input
function a_b = NED_to_BODY(a_n,phi,theta,psi,p,q,r,d)
%#codegen
sphi = sin(phi); sth = sin(theta); tth = tan(theta);
cphi = cos(phi); cth = cos(theta);

J  =...
    [1 sphi*tth cphi*tth;
    0 cphi -sphi;
    0 sphi/cth cphi/cth];

phi_dot     =   p + q*sphi*sth/cth + r*cphi*sth/cth;
theta_dot   =   q*cphi - r*sphi;
psi_dot     =   q*sphi/cth   +   r*cphi/cth;

J_dot = ...
    [0, cphi*tth*phi_dot + sphi*(1+tth*tth)*theta_dot, -sphi*tth*phi_dot+cphi*(1+tth*tth)*theta_dot;
    0, -sphi*phi_dot, -cphi*phi_dot;
    0, (cphi*cth*phi_dot+sphi*sth*theta_dot)/(cth*cth), (-sphi*cth*phi_dot+cphi*sth*theta_dot)/(cth*cth)];

a_b = J\(a_n - J_dot*[p;q;r]);

== matlab function simulator_model/Controllers/Exact_lin_attitude/linearising control law ==
  data: a_b input; phi input; theta input; psi input; u output; p input; q input; r input; d input; parameters parameter
function u = linearising_control_law(a_b,phi,theta,psi,p,q,r,d,parameters)
%#codegen
cth = cos(theta); sth = sin(theta);
cphi = cos(phi); sphi = sin(phi);

%parameters
%%%%%%%%%%%%%%%%%
m = parameters(1);
g = parameters(2);
rho = parameters(3);
V = parameters(4);
%Thruster placement from CO [m]
lx1 = parameters(5);
ly1 = parameters(6);
ly2 = parameters(7);
lx2 = parameters(8);
ly3 = parameters(9);
lx5 = parameters(10);
ly4 = parameters(11);
lz6 = parameters(12);
%%%
zb = parameters(13);
Xu = parameters(14);
Xu_dot = parameters(15);
Xu_abs_u = parameters(16);
Yv = parameters(17);
Yv_dot = parameters(18);
Yv_abs_v = parameters(19);
Zw = parameters(20);
Zw_dot = parameters(21);
Zw_abs_w = parameters(22);
Kp = parameters(23);
Kp_dot = parameters(24);
Kp_abs_p = parameters(25);
Mq = parameters(26);
Mq_dot = parameters(27);
Mq_abs_q = parameters(28);
Nr = parameters(29);
Nr_dot = parameters(30);
Nr_abs_r = parameters(31);
Ix = parameters(32);
Iy = parameters(33);
Iz = parameters(34);
B = rho*g*V;
W = m*g;
%%%%%%%%%%%%%

M =[...
Ix - Kp_dot, 0, 0;
0, Iy - Mq_dot, 0;
0, 0, Iz - Nr_dot];

C =[...
Mq_dot*q*r - Nr_dot*q*r - q*r*(Iy - Iz);
Nr_dot*p*r - Kp_dot*p*r + p*r*(Ix - Iz);
Kp_dot*p*q - Mq_dot*p*q - p*q*(Ix - Iy)];

D = -[...
    (Kp + Kp_abs_p*abs(p))*p;
    (Mq + Mq_abs_q*abs(q))*q;
    (Nr + Nr_abs_r*abs(r))*r];

gn = [...
    -zb*B*cth*sphi;
    -zb*B*sth;
    0];



tau = M*a_b+C+D+gn;
tau = [0;0;0;tau];

T = [...
    0, 0, 1, 1, 0, 0;
    0, 0, 0, 0, 0, -1;
    -1, -1, 0, 0, -1, 0;
    ly1, -ly2, 0, 0, 0, lz6;
    lx1, lx2, 0, 0, -lx5, 0;
    0, 0, ly3, -ly4, 0, 0];

lookup =[...
  -40.0788   -1.0000
  -40.0337   -0.9500
  -37.5428   -0.9250
  -36.6092   -0.9000
  -35.4971   -0.8750
  -33.7623   -0.8500
  -32.3835   -0.8250
  -31.2263   -0.8000
  -29.9809   -0.7750
  -28.5128   -0.7500
  -27.6234   -0.7250
  -26.5554   -0.7000
  -24.7765   -0.6750
  -23.1751   -0.6500
  -22.1522   -0.6250
  -21.3510   -0.6000
  -19.5280   -0.5750
  -18.4600   -0.5500
  -17.3480   -0.5250
  -16.1025   -0.5000
  -14.6345   -0.4750
  -13.0781   -0.4500
  -12.1877   -0.4250
  -10.9874   -0.4000
  -10.0528   -0.3750
   -8.8966   -0.3500
   -7.7404   -0.3250
   -6.8058   -0.3000
   -6.0497   -0.2750
   -5.1151   -0.2500
   -4.2698   -0.2250
   -3.4696   -0.2000
   -2.7135   -0.1750
   -1.8682   -0.1500
   -1.1121   -0.1250
   -0.5335   -0.1000
   -0.2667   -0.0750
         0         0
    0.5786    0.0750
    1.1121    0.1000
    1.8240    0.1250
    2.5801    0.1500
    3.4255    0.1750
    4.0923    0.2000
    5.1151    0.2250
    6.2272    0.2500
    7.0284    0.2750
    8.2739    0.3000
    9.2526    0.3250
   10.8089    0.3500
   12.2328    0.3750
   13.6558    0.4000
   14.9904    0.4250
   16.4585    0.4500
   17.7039    0.4750
   19.2161    0.5000
   20.5508    0.5250
   21.7521    0.5500
   23.6644    0.5750
   24.7324    0.6000
   26.4221    0.6250
   27.7126    0.6500
   29.6249    0.6750
   31.3156    0.7000
   32.8729    0.7250
   33.8065    0.7500
   34.2517    0.7750
   37.0534    0.8000
   38.6549    0.8250
   39.2776    0.8500
   41.1458    0.8750
   42.9257    0.9000
   44.7938    0.9250
   47.1062    0.9500
   48.0408    0.9750
   49.9531    1.0000];
    temp = T\tau;
    for i=1:6
        if temp(i) > 49.9531
            temp(i) = 49.9531;
        elseif temp(i) < -40.0337
            temp(i) = -40.0337;
        end
    end

u = interp1(lookup(:,1),lookup(:,2),temp);

== matlab function simulator_model/Controllers/global_to_local + thrust_alloc/thrust alloc ==
  data: u_b input; u_alloc output size=6
function u_alloc  =...
    thrust_alloc(u_b)
% thrust_allocation = (T.')*inv(T*(T.'));

thrust_allocation = [...
         0    0.5000   -0.2500    0.5000    0.2500         0;
         0   -0.5000   -0.2500   -0.5000    0.2500         0;
    0.5000         0         0         0         0    0.5000;
    0.5000         0         0         0         0   -0.5000;
         0         0   -0.5000         0   -0.5000         0;
         0   -1.0000         0         0         0         0];


u_alloc = thrust_allocation*u_b;

end
